simulink model "Brain"  (R2015a)
settings: Solver=ode45  StartTime=0.0  StopTime=10.0  RelTol=1e-3
settings Model: Creator=Admin  LastModifiedBy=Admin

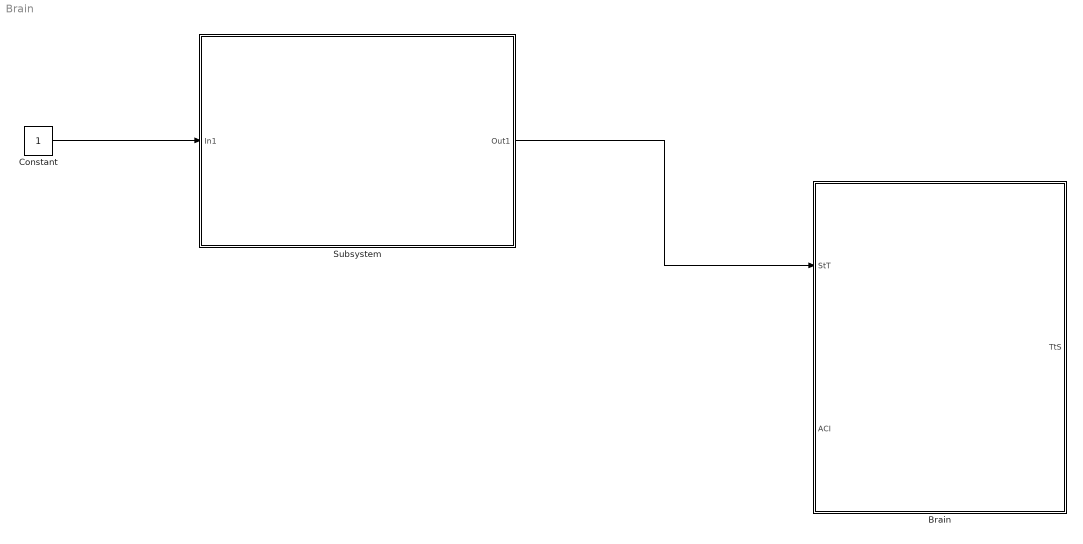
== system Brain ==
  Brain : Stateflow chart  TreatAsAtomicUnit=on
  Constant : Constant
  Subsystem : Subsystem
  wires:
  Subsystem/1(Out1) -> Brain/1(StT)
  Constant/1 -> Subsystem/1(In1)

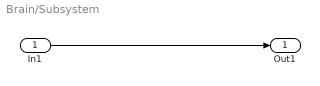
== system Brain/Subsystem ==
  In1 : Inport
  Out1 : Outport
  wires:
  In1/1 -> Out1/1

== stateflow chart Brain/Brain ==
  state Idle
    %Leonie steht rum
    en:
    Test=0
  state SearchForChat
    %Leonie fährt zufällig 100s bis um Person zu finden
  state 3
  (default) -> Idle
  3 -> Idle [order 1] : t>=10
  Idle -> SearchForChat : [test < bla]
  SearchForChat -> 3 : timer > 100
  3 -> 3 [order 2] : t<10
  data: StT input; TtS output; ACI input double
